simulink model "bh_a_spring_mass_model"  (R2018a)
settings: Solver=ode45  StartTime=0.0  StopTime=10.0  RelTol=1e-7
values from neighbouring files (symbols this model uses):
  c = 5    [bh_smd_params.m]
  k = 25    [bh_smd_params.m]
  m = 1    [bh_smd_params.m]
settings Model: Creator=bhorton  LastModifiedBy=bhorton
settings CodeAppCC: StateflowObjectComments=on

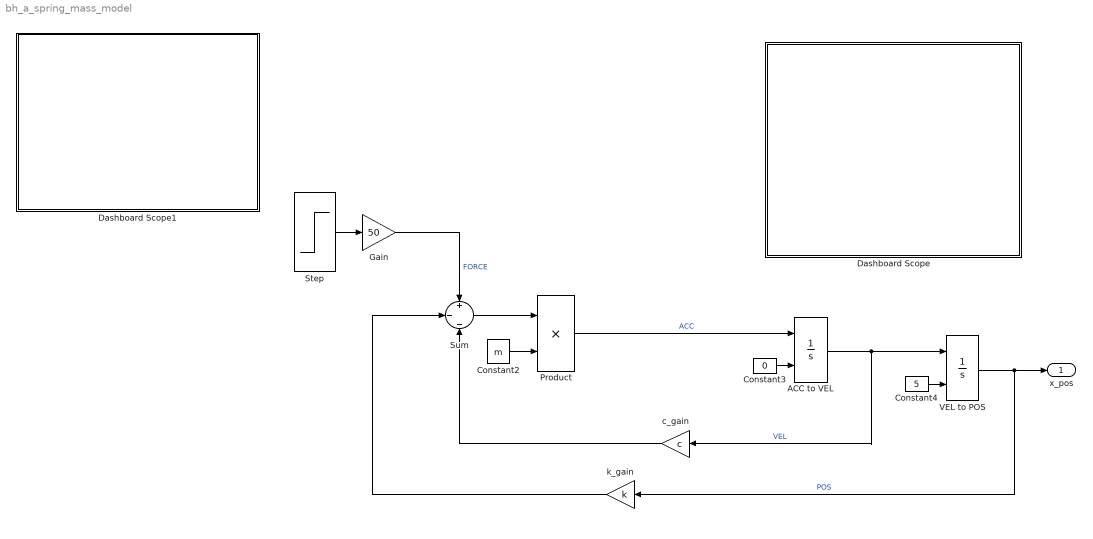
== system bh_a_spring_mass_model ==
  ACC to VEL : Integrator  InitialConditionSource=external
  Constant2 : Constant  Value=m
  Constant3 : Constant  Value=0
  Constant4 : Constant  Value=5
  Dashboard Scope : Subsystem  DialogController=hmiCreateDDGDialog  IsWebBlock=on  mask(MWDashboardBlock){webBlockId=47d7a76a-e090-4f37-bb13-c45fee118520, webBlockType=sdiscope, ShowInitialText=on, HMISrcModelName=bh_a_spring_mass_model}
      mask prompts: webBlockId "WebBlock Id"; webBlockType "WebBlock Type"; HMISrcModelName "Source Model"
      mask help: SimulinkHMI:dialogs:HMIScopeDialogDesc
      mask Help: helpview([docroot '/mapfiles/simulink.map'], 'hmi_scope')
      mask Display:
      | if strcmp(get_param(bdroot(gcb),'BlockDiagramType'), 'library')
      |     image([(matlabroot) '/toolbox/simulink/hmi/icons/DashboardScope.png']);
      | end
  Dashboard Scope1 : Subsystem  DialogController=hmiCreateDDGDialog  IsWebBlock=on  mask(MWDashboardBlock){webBlockId=8ddedbd7-6b40-4d71-b8ad-862d34055e22, webBlockType=sdiscope, ShowInitialText=on, HMISrcModelName=bh_a_spring_mass_model}
      mask prompts: webBlockId "WebBlock Id"; webBlockType "WebBlock Type"; HMISrcModelName "Source Model"
      mask help: SimulinkHMI:dialogs:HMIScopeDialogDesc
      mask Help: helpview([docroot '/mapfiles/simulink.map'], 'hmi_scope')
      mask Display:
      | if strcmp(get_param(bdroot(gcb),'BlockDiagramType'), 'library')
      |     image([(matlabroot) '/toolbox/simulink/hmi/icons/DashboardScope.png']);
      | end
  Gain : Gain  Gain=50
  Product : Product
  Step : Step  Time=5  SampleTime=0
  Sum : Sum  Inputs=+|-|-
  VEL to POS : Integrator  InitialConditionSource=external
  c_gain : Gain  Gain=c
  k_gain : Gain  Gain=k
  x_pos : Outport
  wires:
  Step/1 -> Gain/1
  Gain/1 -> Sum/1  "FORCE"
  Product/1 -> ACC to VEL/1  "ACC"
  ACC to VEL/1 -> c_gain/1, VEL to POS/1  "VEL"
  VEL to POS/1 -> x_pos/1, k_gain/1  "POS"
  Constant2/1 -> Product/2
  Constant3/1 -> ACC to VEL/2
  Constant4/1 -> VEL to POS/2
  Sum/1 -> Product/1
  c_gain/1 -> Sum/3
  k_gain/1 -> Sum/2

== system bh_a_spring_mass_model/Dashboard Scope ==

== system bh_a_spring_mass_model/Dashboard Scope1 ==
